simulink model "banking_nstm"  (R2018b)
settings: configuration reference "Physics" (kept outside this file)
settings Model: DataDictionary=vehicleparameters_vehdynsim.sldd  Creator=staer  LastModifiedBy=staer

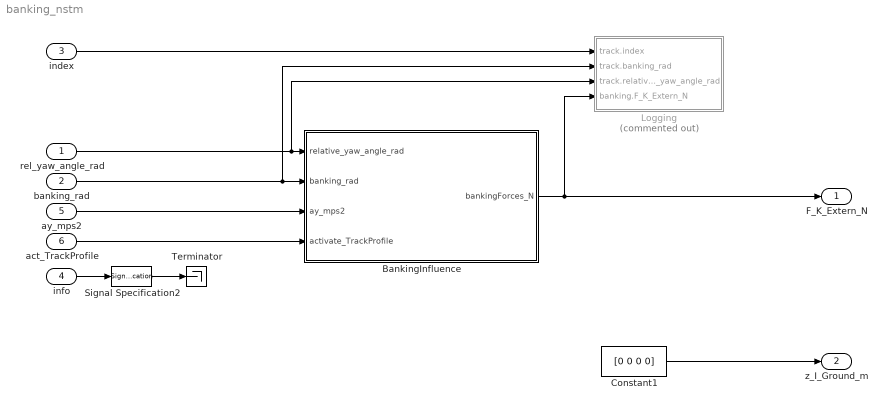
== system banking_nstm ==
  rel_yaw_angle_rad : Inport
  banking_rad : Inport  Port=2
  index : Inport  Port=3
  info : Inport  Port=4
  ay_mps2 : Inport  Port=5
  act_TrackProfile : Inport  Port=6
  BankingInfluence : MATLAB Function  TreatAsAtomicUnit=on
  Constant1 : Constant  Value=[0 0 0 0]
  Logging : Subsystem  Commented=on
  Signal Specification2 : SignalSpecification  Dimensions=[1,4]
  Terminator : Terminator
  F_K_Extern_N : Outport
  z_I_Ground_m : Outport  Port=2
  wires:
  rel_yaw_angle_rad/1 -> Logging/3(track.relative_yaw_angle_rad), BankingInfluence/1(relative_yaw_angle_rad)
  ay_mps2/1 -> BankingInfluence/3(ay_mps2)
  info/1 -> Signal Specification2/1
  index/1 -> Logging/1(track.index)
  BankingInfluence/1(bankingForces_N) -> Logging/4(banking.F_K_Extern_N), F_K_Extern_N/1
  Constant1/1 -> z_I_Ground_m/1
  banking_rad/1 -> BankingInfluence/2(banking_rad), Logging/2(track.banking_rad)
  act_TrackProfile/1 -> BankingInfluence/4(activate_TrackProfile)
  Signal Specification2/1 -> Terminator/1

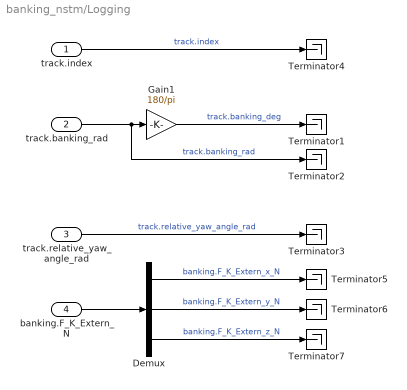
== system banking_nstm/Logging ==
  track.index : Inport
  track.banking_rad : Inport  Port=2
  track.relative_yaw_angle_rad : Inport  Port=3
  banking.F_K_Extern_N : Inport  Port=4
  Demux : Demux  Outputs=3
  Gain1 : Gain  Gain=180/pi
  Terminator{1..7} (7 alike) : Terminator
  wires:
  Gain1/1 -> Terminator1/1  "track.banking_deg"
  track.banking_rad/1 -> Terminator2/1, Gain1/1  "track.banking_rad"
  track.relative_yaw_angle_rad/1 -> Terminator3/1  "track.relative_yaw_angle_rad"
  track.index/1 -> Terminator4/1  "track.index"
  banking.F_K_Extern_N/1 -> Demux/1
  Demux/1 -> Terminator5/1  "banking.F_K_Extern_x_N"
  Demux/2 -> Terminator6/1  "banking.F_K_Extern_y_N"
  Demux/3 -> Terminator7/1  "banking.F_K_Extern_z_N"

== matlab function banking_nstm/BankingInfluence ==
  data: relative_yaw_angle_rad input; banking_rad input; ay_mps2 input; activate_TrackProfile input; bankingForces_N output; VEH__VehicleData__m_Vehicle_kg parameter
function bankingForces_N = fcn(relative_yaw_angle_rad, banking_rad,...
    ay_mps2, activate_TrackProfile, VEH__VehicleData__m_Vehicle_kg)

bankingForces_N = BankingInfluence(relative_yaw_angle_rad, banking_rad,...
    ay_mps2, activate_TrackProfile, VEH__VehicleData__m_Vehicle_kg);
